simulink model "Vehicle_Dyanmic"  (R2023a)
settings: Solver=VariableStepAuto  StartTime=0.0  StopTime=10.0  RelTol=1e-3
values from neighbouring files (symbols this model uses):
  x0 = [0 ... (first row only)    [initVehicleParams.m]
libraries: vrlib x1
settings Model: DataDictionary=vehicleDynamics.sldd  Creator=Julia  LastModifiedBy=Julia

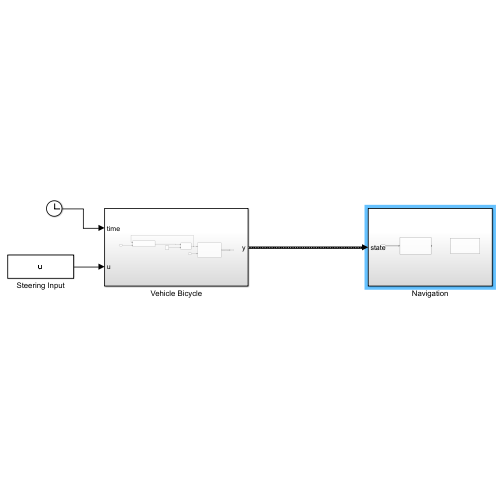
[thumbnail: Simulink's stored preview of the top-level diagram]
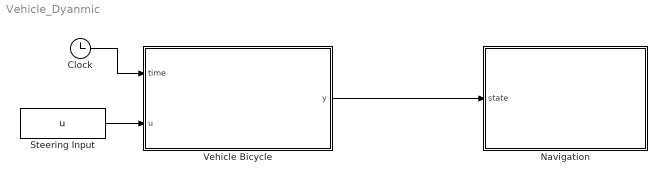
== system Vehicle_Dyanmic ==
  Clock : Clock
  Navigation : Subsystem
  Steering Input : Constant  Value=u
  Vehicle Bicycle : Subsystem
  wires:
  Steering Input/1 -> Vehicle Bicycle/2(u)
  Vehicle Bicycle/1(y) -> Navigation/1(state)
  Clock/1 -> Vehicle Bicycle/1(time)

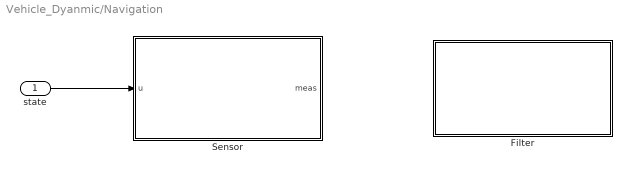
== system Vehicle_Dyanmic/Navigation ==
  state : Inport
  Filter : Subsystem
  "Sensor " : Subsystem
  wires:
  state/1 -> "Sensor "/1(u)

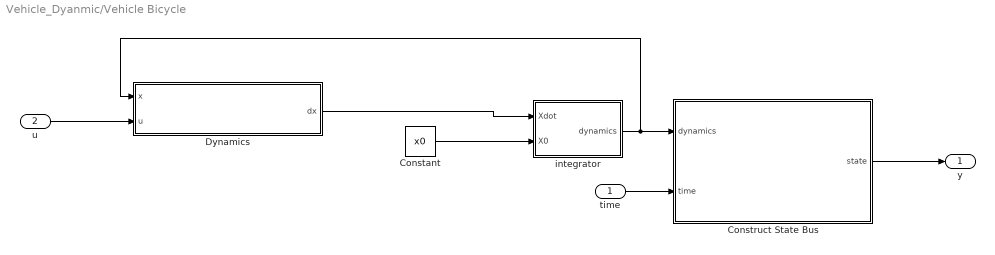
== system Vehicle_Dyanmic/Vehicle Bicycle ==
  time : Inport
  u : Inport  Port=2
  Constant : Constant  Value=x0
  Construct State Bus : Subsystem
  Dynamics : MATLAB Function  TreatAsAtomicUnit=on
  integrator : Subsystem
  y : Outport
  wires:
  u/1 -> Dynamics/2(u)
  Dynamics/1(dx) -> integrator/1(Xdot)
  Constant/1 -> integrator/2(X0)
  time/1 -> Construct State Bus/2(time)
  Construct State Bus/1(state) -> y/1
  integrator/1(dynamics) -> Dynamics/1(x), Construct State Bus/1(dynamics)

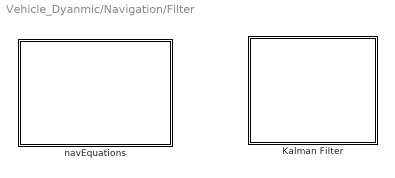
== system Vehicle_Dyanmic/Navigation/Filter ==
  Kalman Filter : Subsystem
  navEquations : Subsystem

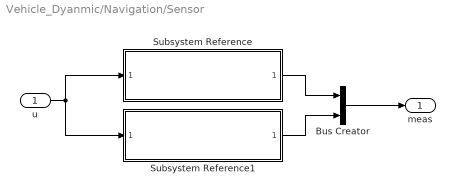
== system Vehicle_Dyanmic/Navigation/Sensor  ==
  u : Inport
  Bus Creator : BusCreator  Inputs=2
  Subsystem Reference : Subsystem  ReferencedSubsystem=IMU
  Subsystem Reference1 : Subsystem  ReferencedSubsystem=Magnetometer
  meas : Outport
  wires:
  u/1 -> Subsystem Reference/1, Subsystem Reference1/1
  Subsystem Reference/1 -> Bus Creator/1
  Subsystem Reference1/1 -> Bus Creator/2
  Bus Creator/1 -> meas/1

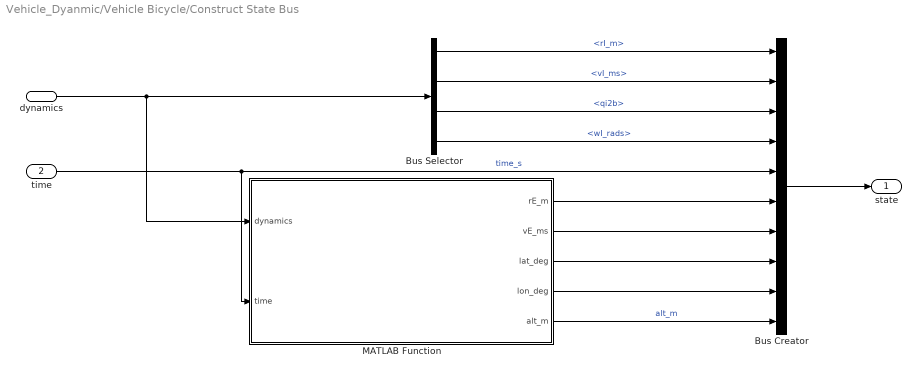
== system Vehicle_Dyanmic/Vehicle Bicycle/Construct State Bus ==
  dynamics : Inport
  time : Inport  Port=2
  Bus Creator : BusCreator  Inputs=10
  Bus Selector : BusSelector  OutputSignals=rI_m,vI_ms,qi2b,wI_rads
  MATLAB Function : MATLAB Function  TreatAsAtomicUnit=on
  state : Outport
      settings: VarSizeSig=Yes
  wires:
  time/1 -> Bus Creator/5, MATLAB Function/2(time)  "time_s"
  Bus Creator/1 -> state/1
  Bus Selector/1 -> Bus Creator/1  "<rI_m>"
  Bus Selector/2 -> Bus Creator/2  "<vI_ms>"
  Bus Selector/3 -> Bus Creator/3  "<qi2b>"
  Bus Selector/4 -> Bus Creator/4  "<wI_rads>"
  MATLAB Function/1(rE_m) -> Bus Creator/6
  MATLAB Function/2(vE_ms) -> Bus Creator/7
  MATLAB Function/3(lat_deg) -> Bus Creator/8
  MATLAB Function/4(lon_deg) -> Bus Creator/9
  MATLAB Function/5(alt_m) -> Bus Creator/10  "alt_m"
  dynamics/1 -> MATLAB Function/1(dynamics), Bus Selector/1

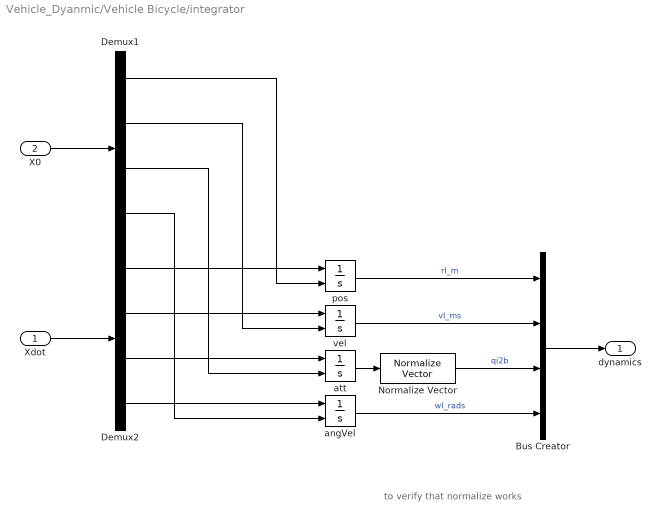
== system Vehicle_Dyanmic/Vehicle Bicycle/integrator ==
  note: to verify that normalize works
  Xdot : Inport
  X0 : Inport  Port=2
  Bus Creator : BusCreator  Inputs=4
  Demux1 : Demux  Outputs=[3 3 4 3]
  Demux2 : Demux  Outputs=[3 3 4 3]
  Normalize Vector : vrlib/Utilities/Normalize Vector  maxzero=1e-12
  angVel : Integrator  InitialConditionSource=external
  att : Integrator  InitialConditionSource=external
  pos : Integrator  InitialConditionSource=external
  vel : Integrator  InitialConditionSource=external
  dynamics : Outport
  wires:
  Xdot/1 -> Demux2/1
  Demux1/1 -> pos/2
  Demux1/2 -> vel/2
  Demux1/4 -> angVel/2
  Demux1/3 -> att/2
  X0/1 -> Demux1/1
  Demux2/4 -> angVel/1
  Demux2/3 -> att/1
  Demux2/2 -> vel/1
  Demux2/1 -> pos/1
  pos/1 -> Bus Creator/1  "rI_m"
  vel/1 -> Bus Creator/2  "vI_ms"
  angVel/1 -> Bus Creator/4  "wI_rads"
  Normalize Vector/1 -> Bus Creator/3  "qi2b"
  att/1 -> Normalize Vector/1
  Bus Creator/1 -> dynamics/1

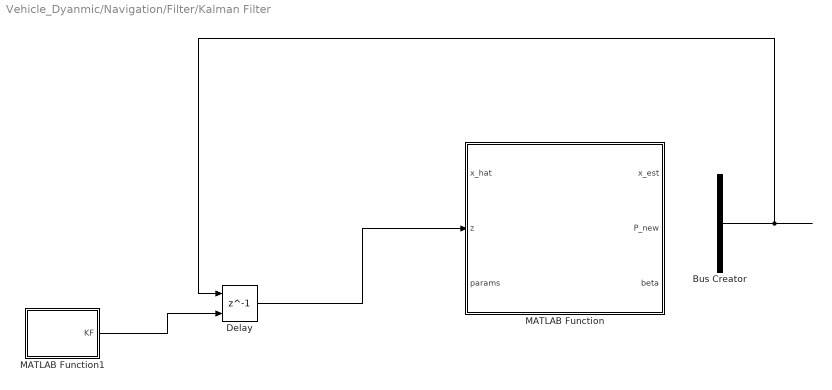
== system Vehicle_Dyanmic/Navigation/Filter/Kalman Filter ==
  Bus Creator : BusCreator  Inputs=3
  Delay : Delay  DelayLength=1  InitialConditionSource=Input port
      settings: InputPortMap=u0,p4
  MATLAB Function : MATLAB Function  TreatAsAtomicUnit=on
  MATLAB Function1 : MATLAB Function  TreatAsAtomicUnit=on
  wires:
  Bus Creator/1 -> Delay/1
  Delay/1 -> MATLAB Function/2(z)
  MATLAB Function1/1(KF) -> Delay/2

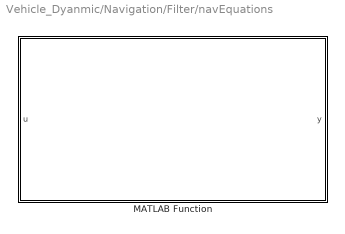
== system Vehicle_Dyanmic/Navigation/Filter/navEquations ==
  MATLAB Function : MATLAB Function  TreatAsAtomicUnit=on

== matlab function Vehicle_Dyanmic/Vehicle Bicycle/Dynamics ==
  data: x input; u input; dx output; params parameter
function dx = BicycleModelDynamics(x, u, params)

dx = BicycleModelDynamics(x, u, params);

== matlab function Vehicle_Dyanmic/Navigation/Filter/Kalman Filter/MATLAB Function ==
  data: x_hat input; z input; x_est output; params input; P_new output; beta output
function [x_est, P_new,beta] = EKF_Bicycle(x_hat, z, params)

[x_est, P_new,beta] = EKF_Bicycle(x_hat, P, z, u, dt, params, R, Q);

== matlab function Vehicle_Dyanmic/Navigation/Filter/Kalman Filter/MATLAB Function1 ==
  data: KF output; params parameter
function KF = fcn(params)

KF = initKF(params)

== matlab function Vehicle_Dyanmic/Navigation/Filter/navEquations/MATLAB Function ==
  data: u input; y output
function y = fcn(u)

y = u;

== matlab function Vehicle_Dyanmic/Vehicle Bicycle/Construct State Bus/MATLAB Function ==
  data: rE_m output; vE_ms output; lat_deg output; lon_deg output; alt_m output; dynamics input; time input; params parameter
function [rE_m,vE_ms,lat_deg,lon_deg,alt_m] = fcn(dynamics,time,params)

% This function calculates all of the common variables that may be used in
% the simulation

rI_m = dynamics.rI_m;
vI_ms = dynamics.vI_ms;

% Inertial to ECEF rotation
wEarth = [0;0;params.Environment.wEarth]; % Earth rotation 
Ci2e = Reci2ecef(params,time);
rE_m = Ci2e*rI_m;
vE_ms = Ci2e*vI_ms - cross(wEarth,rE_m);

[LLA] = ecef2geodetic(rE_m);
lat_deg = LLA(1,:);
lon_deg = LLA(2,:);
alt_m = LLA(3,:);
